simulink model "rapor_301_2_t9"  (R2020a)
settings: Solver=VariableStepAuto  StartTime=0.0  StopTime=100.0  RelTol=1e-3
settings Model: Creator=nartc  LastModifiedBy=nartc

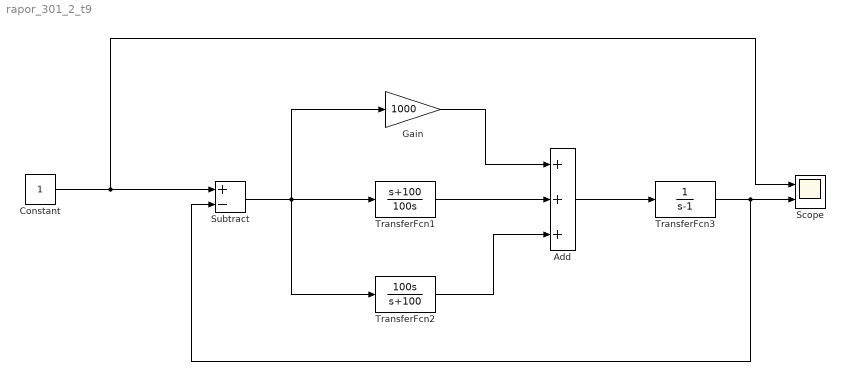
== system rapor_301_2_t9 ==
  Add : Sum  Inputs=+++
  Constant : Constant
  Gain : Gain  Gain=1000
  Scope : Scope  NumInputPorts=2
  Subtract : Sum  Inputs=+-
  TransferFcn1 : TransferFcn  Numerator=[1 100]  Denominator=[100 0]
  TransferFcn2 : TransferFcn  Numerator=[100 0]  Denominator=[1 100]
  TransferFcn3 : TransferFcn  Denominator=[1 -1]
  wires:
  Constant/1 -> Scope/1, Subtract/1
  Subtract/1 -> TransferFcn2/1, Gain/1, TransferFcn1/1
  Gain/1 -> Add/1
  TransferFcn2/1 -> Add/3
  TransferFcn1/1 -> Add/2
  Add/1 -> TransferFcn3/1
  TransferFcn3/1 -> Subtract/2, Scope/2
